simulink library "rw_motor_lib"  (R2016b)
settings: Solver=VariableStepAuto  StartTime=0.0  StopTime=10.0  RelTol=1e-3
undefined symbols (not defined in the file or in its folder): fsw_params
libraries: simulink x1
settings Model: Creator=Taylor  LastModifiedBy=taylorreynolds

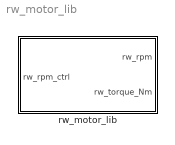
== system rw_motor_lib ==
  rw_motor_lib : Subsystem

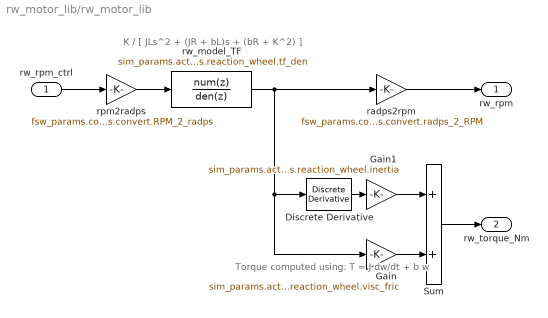
== system rw_motor_lib/rw_motor_lib ==
  note: Torque computed using: T = J dw/dt + b w
  note: K / [ JLs^2 + (JR + bL)s + (bR + K^2) ]
  rw_rpm_ctrl : Inport
  Discrete Derivative : simulink/Discrete/Discrete Derivative  gainval=1.0  ICPrevScaledInput=sim_params.actuators.reaction_wheel.ic.deriv1  OutMin=[]  OutMax=[]  OutDataType=fixdt(1, 16)  OutScaling=2^-10  DoSatur=off
  Gain : Gain  Gain=sim_params.actuators.reaction_wheel.visc_fric
  Gain1 : Gain  Gain=sim_params.actuators.reaction_wheel.inertia
  Sum : Sum
  radps2rpm : Gain  Gain=fsw_params.constants.convert.radps_2_RPM
  rpm2radps : Gain  Gain=fsw_params.constants.convert.RPM_2_radps
  rw_model_TF : DiscreteTransferFcn  Numerator=sim_params.actuators.reaction_wheel.tf_num  Denominator=sim_params.actuators.reaction_wheel.tf_den
  rw_rpm : Outport
  rw_torque_Nm : Outport  Port=2
  wires:
  rw_model_TF/1 -> radps2rpm/1, Gain/1, Discrete Derivative/1
  rw_rpm_ctrl/1 -> rpm2radps/1
  Discrete Derivative/1 -> Gain1/1
  Gain1/1 -> Sum/1
  Gain/1 -> Sum/2
  Sum/1 -> rw_torque_Nm/1
  rpm2radps/1 -> rw_model_TF/1
  radps2rpm/1 -> rw_rpm/1
